simulink model "fuzzy_system_backup"  (R2018b)
settings: Solver=VariableStepAuto  StartTime=0.0  StopTime=10  RelTol=1e-3
undefined symbols (not defined in the file or in its folder): tanks_system
libraries: simulink x1
settings Model: Creator=fredericovaz  LastModifiedBy=fred

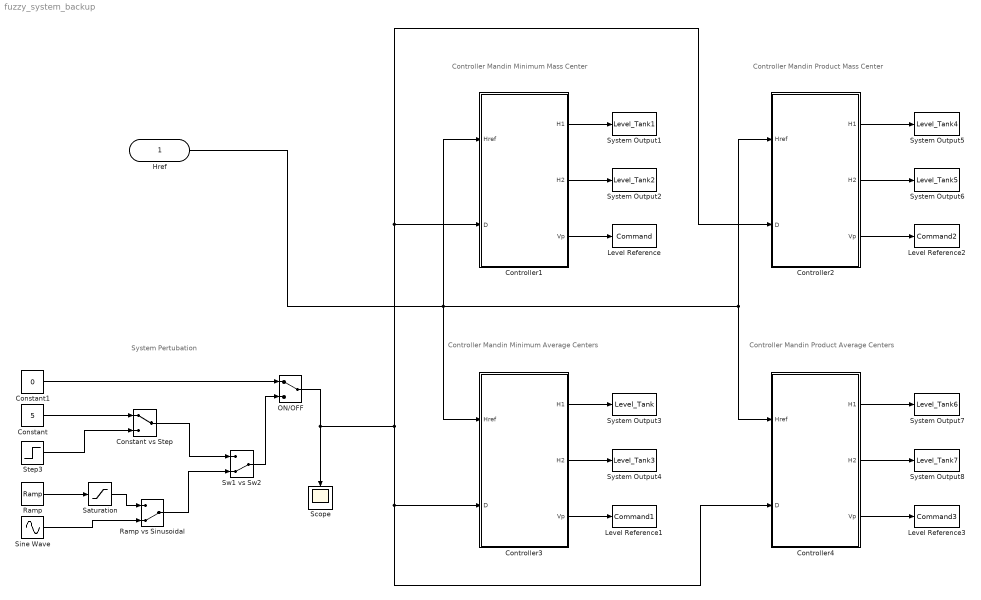
== system fuzzy_system_backup ==
  note: Controller Mandin Minimum Mass Center
  note: Controller Mandin Product Mass Center
  note: Controller Mandin Minimum Average Centers
  note: Controller Mandin Product Average Centers
  note: System Pertubation
  Href : Inport
  Constant : Constant  Value=5
  Constant vs Step : ManualSwitch
  Constant1 : Constant  Value=0
  Controller1 : Subsystem
  Controller2 : Subsystem
  Controller3 : Subsystem
  Controller4 : Subsystem
  Level Reference : ToWorkspace  VariableName=Command  SaveFormat=Timeseries  SampleTime=-1
  Level Reference1 : ToWorkspace  VariableName=Command1  SaveFormat=Timeseries  SampleTime=-1
  Level Reference2 : ToWorkspace  VariableName=Command2  SaveFormat=Timeseries  SampleTime=-1
  Level Reference3 : ToWorkspace  VariableName=Command3  SaveFormat=Timeseries  SampleTime=-1
  ON/OFF : ManualSwitch
  Ramp : simulink/Sources/Ramp  slope=2  start=60  InitialOutput=0
  Ramp vs Sinusoidal : ManualSwitch  CurrentSetting=0
  Saturation : Saturate  UpperLimit=5  LowerLimit=0
  Scope : Scope
  Sine Wave : Sin  Amplitude=5  Frequency=20  SampleTime=0
  Step3 : Step  Time=60  After=5  SampleTime=0
  Sw1 vs Sw2 : ManualSwitch  CurrentSetting=0
  System Output1 : ToWorkspace  VariableName=Level_Tank1  SaveFormat=Timeseries  SampleTime=-1
  System Output2 : ToWorkspace  VariableName=Level_Tank2  SaveFormat=Timeseries  SampleTime=-1
  System Output3 : ToWorkspace  VariableName=Level_Tank  SaveFormat=Timeseries  SampleTime=-1
  System Output4 : ToWorkspace  VariableName=Level_Tank3  SaveFormat=Timeseries  SampleTime=-1
  System Output5 : ToWorkspace  VariableName=Level_Tank4  SaveFormat=Timeseries  SampleTime=-1
  System Output6 : ToWorkspace  VariableName=Level_Tank5  SaveFormat=Timeseries  SampleTime=-1
  System Output7 : ToWorkspace  VariableName=Level_Tank6  SaveFormat=Timeseries  SampleTime=-1
  System Output8 : ToWorkspace  VariableName=Level_Tank7  SaveFormat=Timeseries  SampleTime=-1
  wires:
  Href/1 -> Controller3/1(Href), Controller1/1(Href), Controller2/1(Href), Controller4/1(Href)
  Controller1/2(H2) -> System Output2/1
  Controller1/3(Vp) -> Level Reference/1
  Controller1/1(H1) -> System Output1/1
  Controller3/3(Vp) -> Level Reference1/1
  Controller3/1(H1) -> System Output3/1
  Controller3/2(H2) -> System Output4/1
  Controller2/3(Vp) -> Level Reference2/1
  Controller4/2(H2) -> System Output8/1
  Controller2/2(H2) -> System Output6/1
  Controller2/1(H1) -> System Output5/1
  Controller4/3(Vp) -> Level Reference3/1
  Controller4/1(H1) -> System Output7/1
  ON/OFF/1 -> Scope/1, Controller2/2(D), Controller1/2(D), Controller3/2(D), Controller4/2(D)
  Saturation/1 -> Ramp vs Sinusoidal/1
  Constant/1 -> Constant vs Step/1
  Ramp vs Sinusoidal/1 -> Sw1 vs Sw2/2
  Constant vs Step/1 -> Sw1 vs Sw2/1
  Sine Wave/1 -> Ramp vs Sinusoidal/2
  Step3/1 -> Constant vs Step/2
  Ramp/1 -> Saturation/1
  Constant1/1 -> ON/OFF/1
  Sw1 vs Sw2/1 -> ON/OFF/2

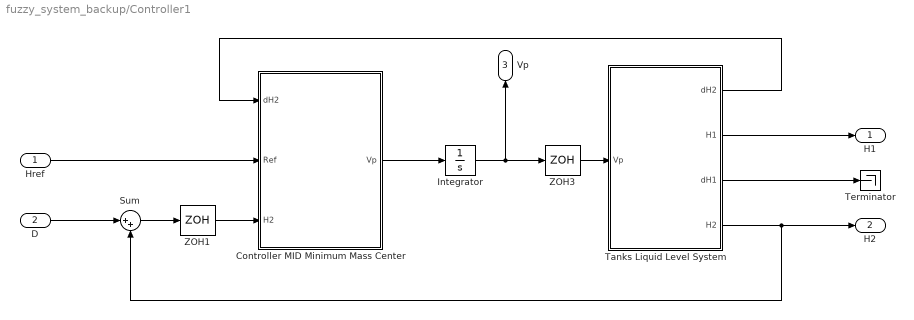
== system fuzzy_system_backup/Controller1 ==
  Href : Inport
  D : Inport  Port=2
  Controller MID Minimum Mass Center : MATLAB Function  TreatAsAtomicUnit=on
  Integrator : Integrator
  Sum : Sum  Inputs=|++
  Tanks Liquid Level System : Subsystem
  Terminator : Terminator
  ZOH1 : ZeroOrderHold  SampleTime=1e-3
  ZOH3 : ZeroOrderHold  SampleTime=1e-3
  H1 : Outport
  H2 : Outport  Port=2
  Vp : Outport  Port=3
  wires:
  Tanks Liquid Level System/4(H2) -> H2/1, Sum/2
  Tanks Liquid Level System/1(dH2) -> Controller MID Minimum Mass Center/1(dH2)
  Href/1 -> Controller MID Minimum Mass Center/2(Ref)
  Tanks Liquid Level System/2(H1) -> H1/1
  D/1 -> Sum/1
  ZOH3/1 -> Tanks Liquid Level System/1(Vp)
  ZOH1/1 -> Controller MID Minimum Mass Center/3(H2)
  Sum/1 -> ZOH1/1
  Integrator/1 -> Vp/1, ZOH3/1
  Controller MID Minimum Mass Center/1(Vp) -> Integrator/1
  Tanks Liquid Level System/3("dH1 ") -> Terminator/1

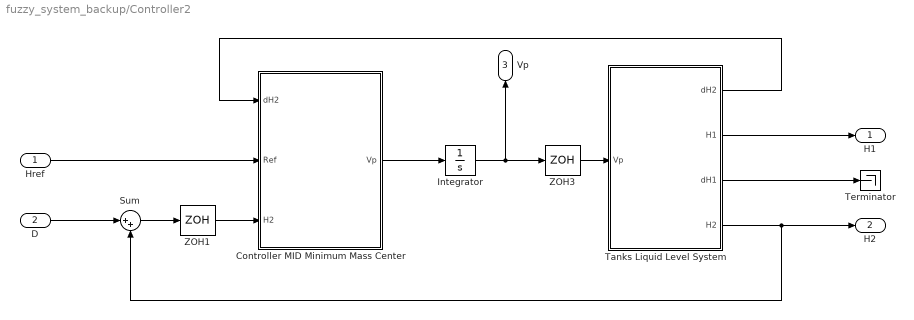
== system fuzzy_system_backup/Controller2 ==
  Href : Inport
  D : Inport  Port=2
  Controller MID Minimum Mass Center : MATLAB Function  TreatAsAtomicUnit=on
  Integrator : Integrator
  Sum : Sum  Inputs=|++
  Tanks Liquid Level System : Subsystem
  Terminator : Terminator
  ZOH1 : ZeroOrderHold  SampleTime=1e-3
  ZOH3 : ZeroOrderHold  SampleTime=1e-3
  H1 : Outport
  H2 : Outport  Port=2
  Vp : Outport  Port=3
  wires:
  Tanks Liquid Level System/4(H2) -> H2/1, Sum/2
  Tanks Liquid Level System/1(dH2) -> Controller MID Minimum Mass Center/1(dH2)
  Href/1 -> Controller MID Minimum Mass Center/2(Ref)
  Tanks Liquid Level System/2(H1) -> H1/1
  D/1 -> Sum/1
  ZOH3/1 -> Tanks Liquid Level System/1(Vp)
  ZOH1/1 -> Controller MID Minimum Mass Center/3(H2)
  Sum/1 -> ZOH1/1
  Integrator/1 -> Vp/1, ZOH3/1
  Controller MID Minimum Mass Center/1(Vp) -> Integrator/1
  Tanks Liquid Level System/3("dH1 ") -> Terminator/1

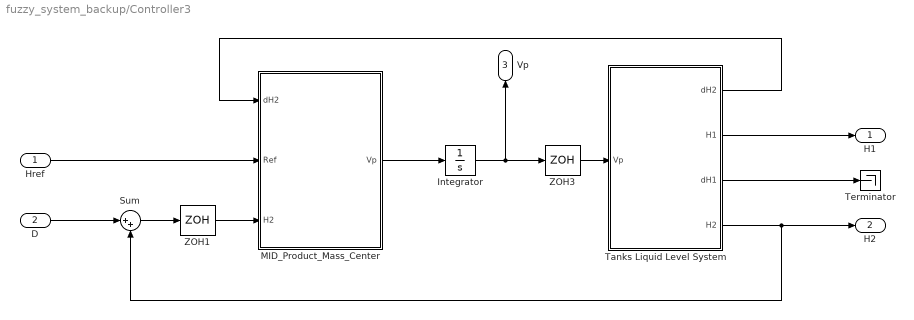
== system fuzzy_system_backup/Controller3 ==
  Href : Inport
  D : Inport  Port=2
  Integrator : Integrator
  MID_Product_Mass_Center : MATLAB Function  TreatAsAtomicUnit=on
  Sum : Sum  Inputs=|++
  Tanks Liquid Level System : Subsystem
  Terminator : Terminator
  ZOH1 : ZeroOrderHold  SampleTime=1e-3
  ZOH3 : ZeroOrderHold  SampleTime=1e-3
  H1 : Outport
  H2 : Outport  Port=2
  Vp : Outport  Port=3
  wires:
  Tanks Liquid Level System/4(H2) -> H2/1, Sum/2
  Tanks Liquid Level System/1(dH2) -> MID_Product_Mass_Center/1(dH2)
  Href/1 -> MID_Product_Mass_Center/2(Ref)
  Tanks Liquid Level System/2(H1) -> H1/1
  D/1 -> Sum/1
  ZOH3/1 -> Tanks Liquid Level System/1(Vp)
  ZOH1/1 -> MID_Product_Mass_Center/3(H2)
  Sum/1 -> ZOH1/1
  Integrator/1 -> Vp/1, ZOH3/1
  MID_Product_Mass_Center/1(Vp) -> Integrator/1
  Tanks Liquid Level System/3("dH1 ") -> Terminator/1

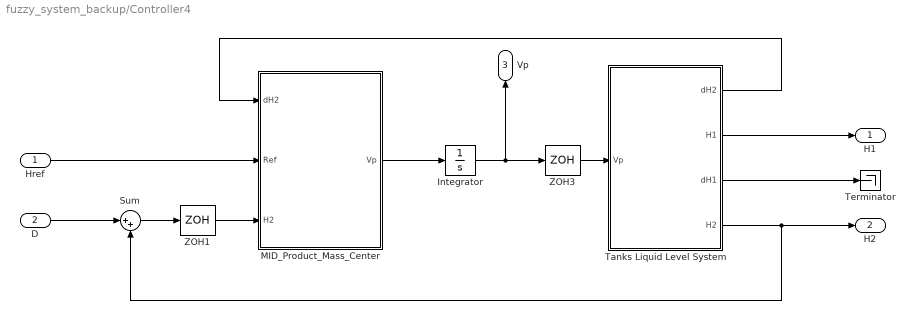
== system fuzzy_system_backup/Controller4 ==
  Href : Inport
  D : Inport  Port=2
  Integrator : Integrator
  MID_Product_Mass_Center : MATLAB Function  TreatAsAtomicUnit=on
  Sum : Sum  Inputs=|++
  Tanks Liquid Level System : Subsystem
  Terminator : Terminator
  ZOH1 : ZeroOrderHold  SampleTime=1e-3
  ZOH3 : ZeroOrderHold  SampleTime=1e-3
  H1 : Outport
  H2 : Outport  Port=2
  Vp : Outport  Port=3
  wires:
  Tanks Liquid Level System/4(H2) -> H2/1, Sum/2
  Tanks Liquid Level System/1(dH2) -> MID_Product_Mass_Center/1(dH2)
  Href/1 -> MID_Product_Mass_Center/2(Ref)
  Tanks Liquid Level System/2(H1) -> H1/1
  D/1 -> Sum/1
  ZOH3/1 -> Tanks Liquid Level System/1(Vp)
  ZOH1/1 -> MID_Product_Mass_Center/3(H2)
  Sum/1 -> ZOH1/1
  Integrator/1 -> Vp/1, ZOH3/1
  MID_Product_Mass_Center/1(Vp) -> Integrator/1
  Tanks Liquid Level System/3("dH1 ") -> Terminator/1

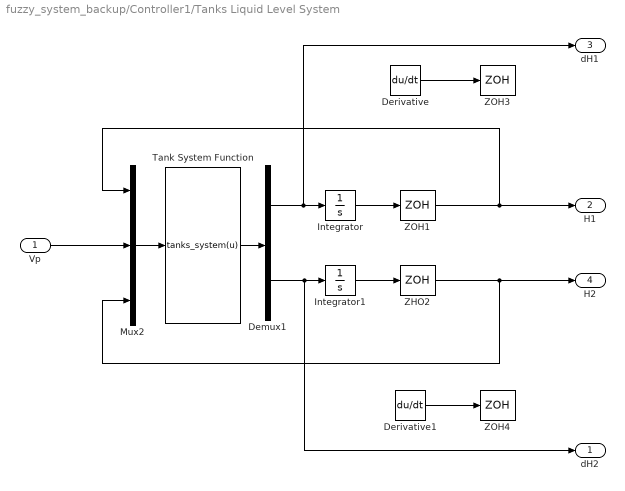
== system fuzzy_system_backup/Controller1/Tanks Liquid Level System ==
  Vp : Inport
  Demux1 : Demux  Outputs=2
  Derivative : Derivative
  Derivative1 : Derivative
  Integrator : Integrator
  Integrator1 : Integrator
  Mux2 : Mux  Inputs=3
  Tank System Function : MATLABFcn  MATLABFcn=tanks_system(u)  OutputDimensions=2
  ZHO2 : ZeroOrderHold  SampleTime=1e-3
  ZOH1 : ZeroOrderHold  SampleTime=1e-3
  ZOH3 : ZeroOrderHold  SampleTime=1e-3
  ZOH4 : ZeroOrderHold  SampleTime=1e-3
  dH2 : Outport
  H1 : Outport  Port=2
  "dH1 " : Outport  Port=3
  H2 : Outport  Port=4
  wires:
  Demux1/2 -> dH2/1, Integrator1/1
  Derivative/1 -> ZOH3/1
  Integrator1/1 -> ZHO2/1
  Vp/1 -> Mux2/2
  ZHO2/1 -> H2/1, Mux2/3
  Integrator/1 -> ZOH1/1
  Derivative1/1 -> ZOH4/1
  Tank System Function/1 -> Demux1/1
  ZOH1/1 -> H1/1, Mux2/1
  Demux1/1 -> "dH1 "/1, Integrator/1
  Mux2/1 -> Tank System Function/1

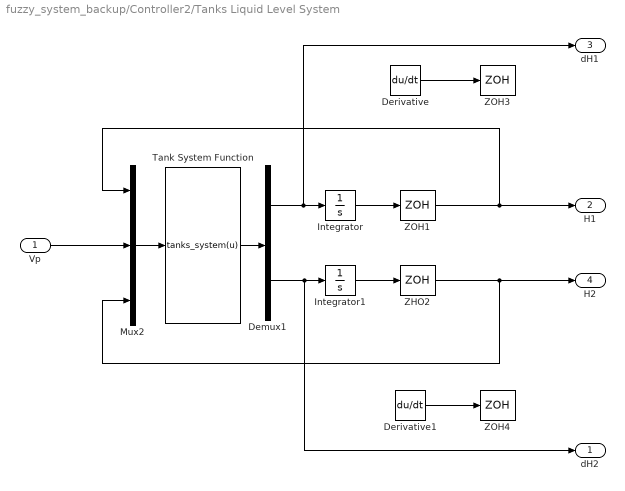
== system fuzzy_system_backup/Controller2/Tanks Liquid Level System ==
  Vp : Inport
  Demux1 : Demux  Outputs=2
  Derivative : Derivative
  Derivative1 : Derivative
  Integrator : Integrator
  Integrator1 : Integrator
  Mux2 : Mux  Inputs=3
  Tank System Function : MATLABFcn  MATLABFcn=tanks_system(u)  OutputDimensions=2
  ZHO2 : ZeroOrderHold  SampleTime=1e-3
  ZOH1 : ZeroOrderHold  SampleTime=1e-3
  ZOH3 : ZeroOrderHold  SampleTime=1e-3
  ZOH4 : ZeroOrderHold  SampleTime=1e-3
  dH2 : Outport
  H1 : Outport  Port=2
  "dH1 " : Outport  Port=3
  H2 : Outport  Port=4
  wires:
  Demux1/2 -> dH2/1, Integrator1/1
  Derivative/1 -> ZOH3/1
  Integrator1/1 -> ZHO2/1
  Vp/1 -> Mux2/2
  ZHO2/1 -> H2/1, Mux2/3
  Integrator/1 -> ZOH1/1
  Derivative1/1 -> ZOH4/1
  Tank System Function/1 -> Demux1/1
  ZOH1/1 -> H1/1, Mux2/1
  Demux1/1 -> "dH1 "/1, Integrator/1
  Mux2/1 -> Tank System Function/1

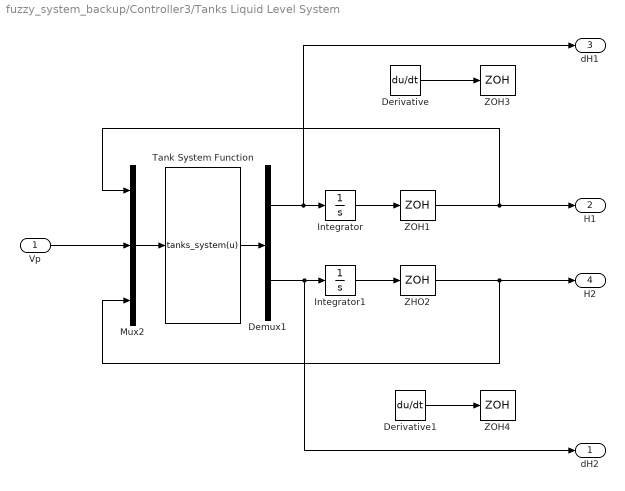
== system fuzzy_system_backup/Controller3/Tanks Liquid Level System ==
  Vp : Inport
  Demux1 : Demux  Outputs=2
  Derivative : Derivative
  Derivative1 : Derivative
  Integrator : Integrator
  Integrator1 : Integrator
  Mux2 : Mux  Inputs=3
  Tank System Function : MATLABFcn  MATLABFcn=tanks_system(u)  OutputDimensions=2
  ZHO2 : ZeroOrderHold  SampleTime=1e-3
  ZOH1 : ZeroOrderHold  SampleTime=1e-3
  ZOH3 : ZeroOrderHold  SampleTime=1e-3
  ZOH4 : ZeroOrderHold  SampleTime=1e-3
  dH2 : Outport
  H1 : Outport  Port=2
  "dH1 " : Outport  Port=3
  H2 : Outport  Port=4
  wires:
  Demux1/2 -> dH2/1, Integrator1/1
  Derivative/1 -> ZOH3/1
  Integrator1/1 -> ZHO2/1
  Vp/1 -> Mux2/2
  ZHO2/1 -> H2/1, Mux2/3
  Integrator/1 -> ZOH1/1
  Derivative1/1 -> ZOH4/1
  Tank System Function/1 -> Demux1/1
  ZOH1/1 -> H1/1, Mux2/1
  Demux1/1 -> "dH1 "/1, Integrator/1
  Mux2/1 -> Tank System Function/1

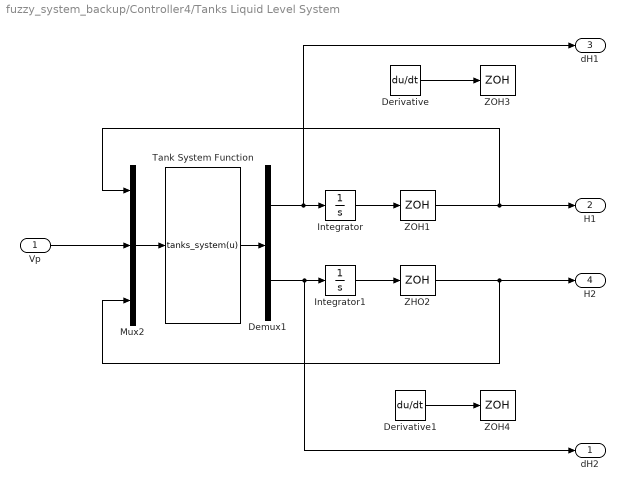
== system fuzzy_system_backup/Controller4/Tanks Liquid Level System ==
  Vp : Inport
  Demux1 : Demux  Outputs=2
  Derivative : Derivative
  Derivative1 : Derivative
  Integrator : Integrator
  Integrator1 : Integrator
  Mux2 : Mux  Inputs=3
  Tank System Function : MATLABFcn  MATLABFcn=tanks_system(u)  OutputDimensions=2
  ZHO2 : ZeroOrderHold  SampleTime=1e-3
  ZOH1 : ZeroOrderHold  SampleTime=1e-3
  ZOH3 : ZeroOrderHold  SampleTime=1e-3
  ZOH4 : ZeroOrderHold  SampleTime=1e-3
  dH2 : Outport
  H1 : Outport  Port=2
  "dH1 " : Outport  Port=3
  H2 : Outport  Port=4
  wires:
  Demux1/2 -> dH2/1, Integrator1/1
  Derivative/1 -> ZOH3/1
  Integrator1/1 -> ZHO2/1
  Vp/1 -> Mux2/2
  ZHO2/1 -> H2/1, Mux2/3
  Integrator/1 -> ZOH1/1
  Derivative1/1 -> ZOH4/1
  Tank System Function/1 -> Demux1/1
  ZOH1/1 -> H1/1, Mux2/1
  Demux1/1 -> "dH1 "/1, Integrator/1
  Mux2/1 -> Tank System Function/1

== matlab function fuzzy_system_backup/Controller3/MID_Product_Mass_Center ==
  data: dH2 input; Ref input; Vp output; H2 input

%%

function Vp  = fcn(dH2, Ref, H2)






y = u;

end

== matlab function fuzzy_system_backup/Controller1/Controller MID Minimum Mass Center ==
  data: dH2 input; Ref input; Vp output; H2 input

%%

function Vp  = fcn(dH2, Ref, H2)






y = u;

end

== matlab function fuzzy_system_backup/Controller2/Controller MID Minimum Mass Center ==
  data: dH2 input; Ref input; Vp output; H2 input

%%

function Vp  = fcn(dH2, Ref, H2)






y = u;

end

== matlab function fuzzy_system_backup/Controller4/MID_Product_Mass_Center ==
  data: dH2 input; Ref input; Vp output; H2 input

%%

function Vp  = fcn(dH2, Ref, H2)






y = u;

end
